simulink model "RobotX_September11"  (R2014a)
settings: Solver=FixedStepDiscrete  StartTime=0.0  StopTime=inf  FixedStep=.1  RelTol=1e-3
undefined symbols (not defined in the file): Com1, Com2, Com3, Com4, DiscIntNeverNeededParam
libraries: xpcseriallib x8, simulink x2, speedgoatlib_IO102 x1, slrtlib x1
(part 2 of 2)

== matlab function RobotX_September11/Main FSM/Gate/Gate ==
  data: Finished output; time input; Valid output; X input; Y input; Psi input; Dist input; Angles input; pts output
function [Finished, Valid, pts] = Gate(time,X,Y,Psi,Dist,Angles)
%Written by Anderson Lebbad on August 9, 2014
%Last Edited by:

%This function sends a forward trajectory (from the initial heading read
%into it) until a landmark is found. Once the landmark is found, a
%trajectory is written to dodge around it.

persistent HeldHeading Found finPt sample
if isempty(HeldHeading)
    HeldHeading = Psi;
    Found = 0;
    finPt = [0 0];
    sample = 50;
end

ts = 5;
dodgeLength = 15;
dodgeWidth = 5;
Finished = 0;
Valid = 0;
pts = zeros(4,2);
%Distance to object in meters
DistM = Dist/100;

%Set Valid bit. If it has been found in a previous timestep, the point is
%invalid, otherwise it is valid every increment of ts or if an object is
%found

%If no Landmark is found, navigate forward
if Found == 0
    %Initial pt
    pts(1,1) = X + 5*cos(HeldHeading*pi/180);
    pts(1,2) = Y + 5*sin(HeldHeading*pi/180);
    %Nothing found
    if Dist(1) == 0
        pts(2,1) = X + 10*cos(HeldHeading*pi/180);
        pts(2,2) = Y + 10*sin(HeldHeading*pi/180);
        pts(3,1) = X + 15*cos(HeldHeading*pi/180);
        pts(3,2) = Y + 15*sin(HeldHeading*pi/180);
        pts(4,1) = X + 20*cos(HeldHeading*pi/180);
        pts(4,2) = Y + 20*sin(HeldHeading*pi/180);
        %Only flip valid bit every ts (seconds)
        sample = sample + 1;
        if sample >= 50
            Valid = 1;
            sample = 0;
        end
        %Something found
    elseif Dist(2) == 0
        %Absolute Heading of object relative to boat's position
        landmarkHeading = mod((Psi + Angles(1)),360);
        lmHeadingRad = landmarkHeading*pi/180;
        %Navigate to it
        pts(2,1) = X + DistM(1)*cos(lmHeadingRad) - dodgeWidth*sin(lmHeadingRad);
        pts(2,2) = Y + DistM(1)*sin(lmHeadingRad) + dodgeWidth*cos(lmHeadingRad);
        pts(3,1) = X + (DistM(1) + dodgeLength)*cos(lmHeadingRad);
        pts(3,2) = Y + (DistM(1) + dodgeLength)*sin(lmHeadingRad);
        pts(4,1) = X + (DistM(1) + 2*dodgeLength)*cos(lmHeadingRad);
        pts(4,2) = Y + (DistM(1) + 2*dodgeLength)*sin(lmHeadingRad);
        finPt = pts(4,:);
        %Flip valid if found
        Valid = 1;
        %Tag object as having been found
        Found = 1;
    else
        %Absolute Heading of object relative to boat's position
        landmarkHeading1 = mod((Psi + Angles(1)),360);
        lmHeadingRad1 = landmarkHeading1*pi/180;
        landmarkHeading2 = mod((Psi + Angles(2)),360);
        lmHeadingRad2 = landmarkHeading2*pi/180;
        %Landmark locations in NED
        lmX1 = X + DistM(1)*cos(lmHeadingRad1);
        lmY1 = Y + DistM(1)*sin(lmHeadingRad1);
        lmX2 = X + DistM(2)*cos(lmHeadingRad2);
        lmY2 = Y + DistM(2)*sin(lmHeadingRad2);
        %Middle point
        midX = (lmX1 + lmX2) / 2;
        midY = (lmY1 + lmY2) / 2;
        %Navigate to it
        pts(2,1) = midX;
        pts(2,2) = midY;
        %Hold heading and continue from midpoint
        pts(3,1) = midX + 5*cos(HeldHeading*pi/180);
        pts(3,2) = midY + 5*sin(HeldHeading*pi/180);
        pts(4,1) = midX + 10*cos(HeldHeading*pi/180);
        pts(4,2) = midY + 10*sin(HeldHeading*pi/180);
        finPt = pts(4,:);
        %Flip valid if found
        Valid = 1;
        %Tag object as having been found
        Found = 2;
    end
end

if Found == 1
    if Dist(2) ~= 0
        %Absolute Heading of object relative to boat's position
        landmarkHeading1 = mod((Psi + Angles(1)),360);
        lmHeadingRad1 = landmarkHeading1*pi/180;
        landmarkHeading2 = mod((Psi + Angles(2)),360);
        lmHeadingRad2 = landmarkHeading2*pi/180;
        %Landmark locations in NED
        lmX1 = X + DistM(1)*cos(lmHeadingRad1);
        lmY1 = Y + DistM(1)*sin(lmHeadingRad1);
        lmX2 = X + DistM(2)*cos(lmHeadingRad2);
        lmY2 = Y + DistM(2)*sin(lmHeadingRad2);
        %Middle point
        midX = (lmX1 + lmX2) / 2;
        midY = (lmY1 + lmY2) / 2;
        %Navigate to it
        pts(2,1) = midX;
        pts(2,2) = midY;
        %Hold heading and continue from midpoint
        pts(3,1) = midX + 5*cos(HeldHeading*pi/180);
        pts(3,2) = midY + 5*sin(HeldHeading*pi/180);
        pts(4,1) = midX + 10*cos(HeldHeading*pi/180);
        pts(4,2) = midY + 10*sin(HeldHeading*pi/180);
        finPt = pts(4,:);
        %Flip valid if found
        Valid = 1;
        %Tag object as having been found
        Found = 2;
    end
end

%Check to see how far the current pose is from the final point in the
%trajectory
if Found >= 1
range = abs(finPt(1)-X)+abs(finPt(2)-Y);
else
    range = 1000;
end
if range <= 5
    Found = 0;
end

end

== matlab function RobotX_September11/Main FSM/Dodge/Calculate Times ==
  data: pts input; u input; Data output
function Data = calcTimes(pts, u)
%Written by Anderson Lebbad on August 9, 2014
%Last Edited:

%Calculates times for the boat to get to points for a trajectory, and
%formats Data for communication

%Initialize
Data = zeros(12,1);
traj = zeros(4,3);
traj(:,1:2) = pts;



for k = 2:4
    %Calculate distance to travel from last point
    distTravel = sqrt(sum((pts(k-1,:)-pts(k,:)).^2));
    %Assume 1m per second speed
    traj(k,3) = traj(k-1,3) + distTravel;
    %Add time based off initial velocity to get to first point past initial
    if k == 2
        traj(k,3) = traj(k,3) + 2.5*abs(2-u);
    end
end


%Output Data
for i=1:4
    for j = 1:3
        Data(3*(i-1)+j) = traj(i,j);
    end
end

== matlab function RobotX_September11/Main FSM/RCHold/Set Pose ==
  data: X input; Data output; Y input; Psi input
function Data = setPose(X,Y,Psi)
%Written by Anderson Lebbad on August 9, 2014
%Last Edited:

%This function passes the current pose data with a heading offset as the
%desired pose for the station keeping controller to use.

persistent holdPose

if isempty(holdPose)
    holdPose = [X Y Psi];
end

%Initialize Data variable
Data = zeros(12,1);

%Set desired pose
Data(1) = holdPose(1);
Data(2) = holdPose(2);
Data(3) = holdPose(3);

== matlab function RobotX_September11/Main FSM/Termination/Point ==
  data: X input; Data output; Y input; Psi input; Dist input; Angle input
function Data = Point(X,Y,Psi,Dist,Angle)
%Written by Anderson Lebbad on August 9, 2014
%Last Edited:

%This function passes the current pose data with a heading offset as the
%desired pose for the station keeping controller to use.

persistent holdPose

if isempty(holdPose)
    holdPose = [X Y Psi + 180];
end

%Initialize Data variable
Data = zeros(12,1);

if Dist(1) ~= 0
    holdPose(3) = Psi + Angle(1);
end

%Set desired pose
Data(1) = holdPose(1);
Data(2) = holdPose(2);
Data(3) = holdPose(3);

== matlab function RobotX_September11/Main FSM/Gate1/Calculate Times ==
  data: pts input; u input; Data output
function Data = calcTimes(pts, u)
%Written by Anderson Lebbad on August 9, 2014
%Last Edited:

%Calculates times for the boat to get to points for a trajectory, and
%formats Data for communication

%Initialize
Data = zeros(12,1);
traj = zeros(4,3);
traj(:,1:2) = pts;



for k = 2:4
    %Calculate distance to travel from last point
    distTravel = sqrt(sum((pts(k-1,:)-pts(k,:)).^2));
    %Assume 1m per second speed
    traj(k,3) = traj(k-1,3) + distTravel;
    %Add time based off initial velocity to get to first point past initial
    if k == 2
        traj(k,3) = traj(k,3) + 2.5*abs(2-u);
    end
end


%Output Data
for i=1:4
    for j = 1:3
        Data(3*(i-1)+j) = traj(i,j);
    end
end

== matlab function RobotX_September11/Main FSM/Gate1/Gate ==
  data: Finished output; time input; Valid output; X input; Y input; Psi input; Dist input; Angles input; pts output
function [Finished, Valid, pts] = Gate(time,X,Y,Psi,Dist,Angles)
%Written by Anderson Lebbad on August 9, 2014
%Last Edited by:

%This function sends a forward trajectory (from the initial heading read
%into it) until a landmark is found. Once the landmark is found, a
%trajectory is written to dodge around it.

persistent HeldHeading Found finPt sample
if isempty(HeldHeading)
    HeldHeading = Psi;
    Found = 0;
    finPt = [0 0];
    sample = 50;
end

ts = 5;
dodgeLength = 15;
dodgeWidth = 5;
Finished = 0;
Valid = 0;
pts = zeros(4,2);
%Distance to object in meters
DistM = Dist/100;

%Set Valid bit. If it has been found in a previous timestep, the point is
%invalid, otherwise it is valid every increment of ts or if an object is
%found

%If no Landmark is found, navigate forward
if Found == 0
    %Initial pt
    pts(1,1) = X + 5*cos(HeldHeading*pi/180);
    pts(1,2) = Y + 5*sin(HeldHeading*pi/180);
    %Nothing found
    if Dist(1) == 0
        pts(2,1) = X + 10*cos(HeldHeading*pi/180);
        pts(2,2) = Y + 10*sin(HeldHeading*pi/180);
        pts(3,1) = X + 15*cos(HeldHeading*pi/180);
        pts(3,2) = Y + 15*sin(HeldHeading*pi/180);
        pts(4,1) = X + 20*cos(HeldHeading*pi/180);
        pts(4,2) = Y + 20*sin(HeldHeading*pi/180);
        %Only flip valid bit every ts (seconds)
        sample = sample + 1;
        if sample >= 50
            Valid = 1;
            sample = 0;
        end
        %Something found
    elseif Dist(2) == 0
        %Absolute Heading of object relative to boat's position
        landmarkHeading = mod((Psi + Angles(1)),360);
        lmHeadingRad = landmarkHeading*pi/180;
        %Navigate to it
        pts(2,1) = X + DistM(1)*cos(lmHeadingRad) - dodgeWidth*sin(lmHeadingRad);
        pts(2,2) = Y + DistM(1)*sin(lmHeadingRad) + dodgeWidth*cos(lmHeadingRad);
        pts(3,1) = X + (DistM(1) + dodgeLength)*cos(lmHeadingRad);
        pts(3,2) = Y + (DistM(1) + dodgeLength)*sin(lmHeadingRad);
        pts(4,1) = X + (DistM(1) + 2*dodgeLength)*cos(lmHeadingRad);
        pts(4,2) = Y + (DistM(1) + 2*dodgeLength)*sin(lmHeadingRad);
        finPt = pts(4,:);
        %Flip valid if found
        Valid = 1;
        %Tag object as having been found
        Found = 1;
    else
        %Absolute Heading of object relative to boat's position
        landmarkHeading1 = mod((Psi + Angles(1)),360);
        lmHeadingRad1 = landmarkHeading1*pi/180;
        landmarkHeading2 = mod((Psi + Angles(2)),360);
        lmHeadingRad2 = landmarkHeading2*pi/180;
        %Landmark locations in NED
        lmX1 = X + DistM(1)*cos(lmHeadingRad1);
        lmY1 = Y + DistM(1)*sin(lmHeadingRad1);
        lmX2 = X + DistM(2)*cos(lmHeadingRad2);
        lmY2 = Y + DistM(2)*sin(lmHeadingRad2);
        %Middle point
        midX = (lmX1 + lmX2) / 2;
        midY = (lmY1 + lmY2) / 2;
        %Navigate to it
        pts(2,1) = midX;
        pts(2,2) = midY;
        %Hold heading and continue from midpoint
        pts(3,1) = midX + 5*cos(HeldHeading*pi/180);
        pts(3,2) = midY + 5*sin(HeldHeading*pi/180);
        pts(4,1) = midX + 10*cos(HeldHeading*pi/180);
        pts(4,2) = midY + 10*sin(HeldHeading*pi/180);
        finPt = pts(4,:);
        %Flip valid if found
        Valid = 1;
        %Tag object as having been found
        Found = 2;
    end
end

if Found == 1
    if Dist(2) ~= 0
        %Absolute Heading of object relative to boat's position
        landmarkHeading1 = mod((Psi + Angles(1)),360);
        lmHeadingRad1 = landmarkHeading1*pi/180;
        landmarkHeading2 = mod((Psi + Angles(2)),360);
        lmHeadingRad2 = landmarkHeading2*pi/180;
        %Landmark locations in NED
        lmX1 = X + DistM(1)*cos(lmHeadingRad1);
        lmY1 = Y + DistM(1)*sin(lmHeadingRad1);
        lmX2 = X + DistM(2)*cos(lmHeadingRad2);
        lmY2 = Y + DistM(2)*sin(lmHeadingRad2);
        %Middle point
        midX = (lmX1 + lmX2) / 2;
        midY = (lmY1 + lmY2) / 2;
        %Navigate to it
        pts(2,1) = midX;
        pts(2,2) = midY;
        %Hold heading and continue from midpoint
        pts(3,1) = midX + 5*cos(HeldHeading*pi/180);
        pts(3,2) = midY + 5*sin(HeldHeading*pi/180);
        pts(4,1) = midX + 10*cos(HeldHeading*pi/180);
        pts(4,2) = midY + 10*sin(HeldHeading*pi/180);
        finPt = pts(4,:);
        %Flip valid if found
        Valid = 1;
        %Tag object as having been found
        Found = 2;
    end
end

%Check to see how far the current pose is from the final point in the
%trajectory
if Found >= 1
range = abs(finPt(1)-X)+abs(finPt(2)-Y);
else
    range = 1000;
end
if range <= 5
    Found = 0;
end

end

== matlab function RobotX_September11/Main FSM/Approach/Approach ==
  data: Finished output; time input; Valid output; X input; Y input; Psi input; pts output
function [Finished, Valid, pts] = Approach(time,X,Y,Psi)
%Written by Anderson Lebbad on August 9, 2014
%Last Edited by:

%This function sends a forward trajectory (from the initial heading read
%into it) until a landmark is found. Once the landmark is found, a
%trajectory is written to approach it.

persistent HeldHeading startX startY lastTime
if isempty(HeldHeading)
    HeldHeading = Psi;
    startX = X;
    startY = Y;
    lastTime = -5;
end

Finished = 0;
Valid = 0;
pts = zeros(4,2);

%Set Valid bit. If it has been found in a previous timestep, the point is
%invalid, otherwise it is valid every increment of ts or if an object is
%found

%Initial pt
pts(1,1) = X + 5*cos(HeldHeading*pi/180);
pts(1,2) = Y + 5*sin(HeldHeading*pi/180);
pts(2,1) = X + 10*cos(HeldHeading*pi/180);
pts(2,2) = Y + 10*sin(HeldHeading*pi/180);
pts(3,1) = X + 15*cos(HeldHeading*pi/180);
pts(3,2) = Y + 15*sin(HeldHeading*pi/180);
pts(4,1) = X + 20*cos(HeldHeading*pi/180);
pts(4,2) = Y + 20*sin(HeldHeading*pi/180);
%Only flip valid bit every ts (seconds)
timed = time-lastTime;
if timed >= 5
    Valid = 1;
    lastTime = time;
end


%Check to see how far the current pose is from the final point in the
%trajectory
range = abs(X-startX)+abs(Y-startY);
if range > 10
    Finished = 1;
end

end

== matlab function RobotX_September11/Main FSM/Approach/Calculate Times ==
  data: pts input; u input; Data output
function Data = calcTimes(pts, u)
%Written by Anderson Lebbad on August 9, 2014
%Last Edited:

%Calculates times for the boat to get to points for a trajectory, and
%formats Data for communication

%Initialize
Data = zeros(12,1);
traj = zeros(4,3);
traj(:,1:2) = pts;

for k = 2:4
    %Calculate distance to travel from last point
    distTravel = sqrt(sum((pts(k-1,:)-pts(k,:)).^2));
    %Assume 1m per second speed
    traj(k,3) = traj(k-1,3) + distTravel;
    %Add time based off initial velocity to get to first point past initial
    if k == 2
        traj(k,3) = traj(k,3) + 2.5*abs(2-u);
    end
end


%Output Data
for i=1:4
    for j = 1:3
        Data(3*(i-1)+j) = traj(i,j);
    end
end

== matlab function RobotX_September11/Main FSM/Main Task Option/Message Composer ==
  data: taskStrInit input; taskStrAdj output
function taskStrAdj = composeMessage(taskStrInit)
%Written by Anderson Lebbad on August 9, 2013
%Last Edited: Edward Zhu on June 2, 2014

%This function adjusts the length of a vector to a set value by filling
%the remaining space with 0's. This is necessary for data store objects
%that have a fixed size for the memory allocation, but a variable length
%input.

%Length of message packet
strLength = 8;

%Size of text in message
taskStrLength = size(taskStrInit,1);

%Pad end of text with zeros
taskStrAdj = [taskStrInit' zeros(1,strLength-taskStrLength)];

== matlab function RobotX_September11/Parameters/GPS Points/GPS Selector ==
  data: course input; ssGate output; rtnIn input; ssGateA input; transWptA input; obstNavStartA input; obstNavEndA input; acouLocA input; dockA input; ssGateB input; transWptB input; obstNavStartB input; obstNavEndB input; acouLocB input; dockB input; ssGateT input; transWptT input; obstNavStartT input; obstNavEndT input; acouLocT input; dockT input; transWpt output; obstNavStart output; obstNavEnd output; acouLoc output; dock output; rtnOut output
function [ssGate,transWpt,obstNavStart,obstNavEnd,acouLoc,dock,rtnOut] = ...
    GPSselector(course,rtnIn,...
    ssGateA,transWptA,obstNavStartA,obstNavEndA,acouLocA,dockA,...
    ssGateB,transWptB,obstNavStartB,obstNavEndB,acouLocB,dockB,...
    ssGateT,transWptT,obstNavStartT,obstNavEndT,acouLocT,dockT)

%Written by: Anderson Lebbad on July 18, 2013
%Last Edited: Edward Zhu on June
%   Data type mismatch addressed
%   Character conversion redundant

%Selects GPS Points to use based on input Course

%Check value of CourseStr and pass inputs accordingly

switch course
    case uint8('A')
        ssGate = ssGateA;
        transWpt = transWptA;
        obstNavStart = obstNavStartA;
        obstNavEnd = obstNavEndA;
        acouLoc = acouLocA;
        dock = dockA;
        rtnOut = rtnIn;
        
    case uint8('B')
        ssGate = ssGateB;
        transWpt = transWptB;
        obstNavStart = obstNavStartB;
        obstNavEnd = obstNavEndB;
        acouLoc = acouLocB;
        dock = dockB;
        rtnOut = rtnIn;
        
    otherwise
        ssGate = ssGateT;
        transWpt = transWptT;
        obstNavStart = obstNavStartT;
        obstNavEnd = obstNavEndT;
        acouLoc = acouLocT;
        dock = dockT;
        rtnOut = rtnIn;
end
